simulink model "PosCtrl_tune"  (R2020b)
settings: Solver=FixedStepAuto  StartTime=0.0  StopTime=inf  FixedStep=0.01  RelTol=1e-3
InitFcn:
  | Init_control;
values from neighbouring files (symbols this model uses):
  DEG2RAD = 0.0174533    [Init_control.m]
  Kd_PITCH_AngleRate = 0.001    [Init_control.m]
  Kd_ROLL_AngleRate = 0.001    [Init_control.m]
  Kd_YAW_AngleRate = 0.00    (= 0)    [Init_control.m]
  Ki_PITCH_AngleRate = 0.02    [Init_control.m]
  Ki_ROLL_AngleRate = 0.02    [Init_control.m]
  Ki_YAW_AngleRate = 0.01    [Init_control.m]
  Kp_PITCH_ANGLE = 6.5    [Init_control.m]
  Kp_PITCH_AngleRate = 0.1    [Init_control.m]
  Kp_ROLL_ANGLE = 6.5    [Init_control.m]
  Kp_ROLL_AngleRate = 0.1    [Init_control.m]
  Kp_YAW_AngleRate = 0.5    [Init_control.m]
  Kpxp = 1.0    (= 1)    [Init_control.m]
  Kpyp = 1.0    (= 1)    [Init_control.m]
  Kpzp = 4.0    (= 4)    [Init_control.m]
  Kvxd = 0.01    [Init_control.m]
  Kvxi = 0.4    [Init_control.m]
  Kvxp = 2.5    [Init_control.m]
  Kvyd = 0.01    [Init_control.m]
  Kvyi = 0.4    [Init_control.m]
  Kvyp = 2.5    [Init_control.m]
  Kvzd = 0.005    [Init_control.m]
  Kvzi = 0.01    [Init_control.m]
  Kvzp = 0.45    [Init_control.m]
  MAX_CONTROL_ANGLE_PITCH = 35    [Init_control.m]
  MAX_CONTROL_ANGLE_RATE_PITCH = 220    [Init_control.m]
  MAX_CONTROL_ANGLE_RATE_ROLL = 220    [Init_control.m]
  MAX_CONTROL_ANGLE_ROLL = 35    [Init_control.m]
  MAX_CONTROL_VELOCITY_XY = 18    [Init_control.m]
  MAX_CONTROL_VELOCITY_Z = 3    [Init_control.m]
  MAX_MAN_THR = 0.9    [Init_control.m]
  ModelInit_AngEuler = [0, 0, 0]    [Init_control.m]
  ModelInit_PosE = [0, 0, 0]    [Init_control.m]
  ModelInit_Rads = 557.142    [Init_control.m]
  ModelInit_RateB = [0, 0, 0]    [Init_control.m]
  ModelInit_VelB = [0, 0, 0]    [Init_control.m]
  Saturation_I_ah = 3.43    [Init_control.m]
  Saturation_I_az = 5    [Init_control.m]
  Saturation_I_RP_Max = 0.3    [Init_control.m]
  Saturation_I_RP_Min = -0.3    [Init_control.m]
  Saturation_I_Y_Max = 0.2    [Init_control.m]
  Saturation_I_Y_Min = -0.2    [Init_control.m]
  THR_HOVER = 0.609    [Init_control.m]
undefined symbols (not defined in the file or in its folder): DiscIntNeverNeededParam, ModelParam_envGravityAcc, ModelParam_motorCr, ModelParam_motorJm, ModelParam_motorT, ModelParam_motorWb, ModelParam_rotorCm, ModelParam_rotorCt, ModelParam_uavCCm, ModelParam_uavCd, ModelParam_uavJ, ModelParam_uavMass, ModelParam_uavR
libraries: simulink x18, slrealtimeutilitieslib x7, dspnetwork x7, sharedutil x6, aerolibanimutils x1
(part 3 of 3)

== matlab function PosCtrl_tune/01/Quadcopter Dynamics/六自由度模型/Rigid-Body Kinematic Model /Quaternion to Euler ==
  data: q input; y output
function y = fcn(q)
 %Function description:
%  Quaternions to Euler
phi = atan2(2*(q(1)*q(2) + q(3)*q(4)), (1 - 2*(q(2)*q(2) + q(3)*q(3))));
theta = asin(2*(q(1)*q(3) - q(2)*q(4)));
psi = atan2(2*(q(1)*q(4) + q(2)*q(3)), (1 - 2*(q(3)*q(3) + q(4)*q(4))));
y = [phi theta psi];

== matlab function PosCtrl_tune/01/Quadcopter Dynamics/六自由度模型/Rigid-Body Kinematic Model /Quaternion to rotation matrix ==
  data: q input; Reb output
function Reb = fcn(q)
%Function description;
%  The rotation matrix of the Aircraft-Body Coordinate Frame (ABCF) to the
%  Earth-Fixed Coordinate Frame (EFCF) is obtained from the quaternions
Reb = [q(1)*q(1) + q(2)*q(2) - q(3)*q(3) - q(4)*q(4), 2*(q(2)*q(3) - q(1)*q(4)), 2*(q(2)*q(4) + q(1)*q(3))
           2*(q(2)*q(3) + q(1)*q(4)), q(1)*q(1) - q(2)*q(2) + q(3)*q(3) - q(4)*q(4), 2*(q(3)*q(4) - q(1)*q(2))
           2*(q(2)*q(4) - q(1)*q(3)), 2*(q(3)*q(4) + q(1)*q(2)), q(1)*q(1) - q(2)*q(2) - q(3)*q(3) + q(4)*q(4)];

== matlab function PosCtrl_tune/01/Quadcopter Dynamics/六自由度模型/Rigid-Body Kinematic Model /Quaternions model ==
  data: pqr input; qdot output; q input
function qdot = fcn(pqr, q)
%Function description:
%  Quaternions model
qdot = 0.5*[0, -pqr(1), -pqr(2), -pqr(3); pqr(1), 0, pqr(3), -pqr(2); pqr(2), -pqr(3), 0, pqr(1); pqr(3), pqr(2), -pqr(1), 0]*q;

== matlab function PosCtrl_tune/00/Quadcopter Dynamics/六自由度模型/Rigid-Body Kinematic Model /Quaternion to rotation matrix ==
  data: q input; Reb output
function Reb = fcn(q)
%Function description;
%  The rotation matrix of the Aircraft-Body Coordinate Frame (ABCF) to the
%  Earth-Fixed Coordinate Frame (EFCF) is obtained from the quaternions
Reb = [q(1)*q(1) + q(2)*q(2) - q(3)*q(3) - q(4)*q(4), 2*(q(2)*q(3) - q(1)*q(4)), 2*(q(2)*q(4) + q(1)*q(3))
           2*(q(2)*q(3) + q(1)*q(4)), q(1)*q(1) - q(2)*q(2) + q(3)*q(3) - q(4)*q(4), 2*(q(3)*q(4) - q(1)*q(2))
           2*(q(2)*q(4) - q(1)*q(3)), 2*(q(3)*q(4) + q(1)*q(2)), q(1)*q(1) - q(2)*q(2) - q(3)*q(3) + q(4)*q(4)];

== matlab function PosCtrl_tune/00/Quadcopter Dynamics/六自由度模型/Rigid-Body Kinematic Model /Quaternion to Euler ==
  data: q input; y output
function y = fcn(q)
 %Function description:
%  Quaternions to Euler
phi = atan2(2*(q(1)*q(2) + q(3)*q(4)), (1 - 2*(q(2)*q(2) + q(3)*q(3))));
theta = asin(2*(q(1)*q(3) - q(2)*q(4)));
psi = atan2(2*(q(1)*q(4) + q(2)*q(3)), (1 - 2*(q(3)*q(3) + q(4)*q(4))));
y = [phi theta psi];
